simulink model "Modelo_global_NL_control_sobre_eje_q_2_c_VI"  (R2017a)
settings: Solver=VariableStepAuto  StartTime=0.0  StopTime=10.0  RelTol=1e-3
undefined symbols (not defined in the file): alfa_cu, beq, Cts, Jeq, LambdaM, Ld, Lq, Pp, Rs, Rsref, Rts, Tamb, Tsref
settings Model: Creator=merem  LastModifiedBy=merem

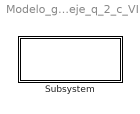
== system Modelo_global_NL_control_sobre_eje_q_2_c_VI ==
  Subsystem : Subsystem

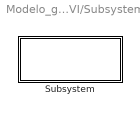
== system Modelo_global_NL_control_sobre_eje_q_2_c_VI/Subsystem ==
  Subsystem : Subsystem

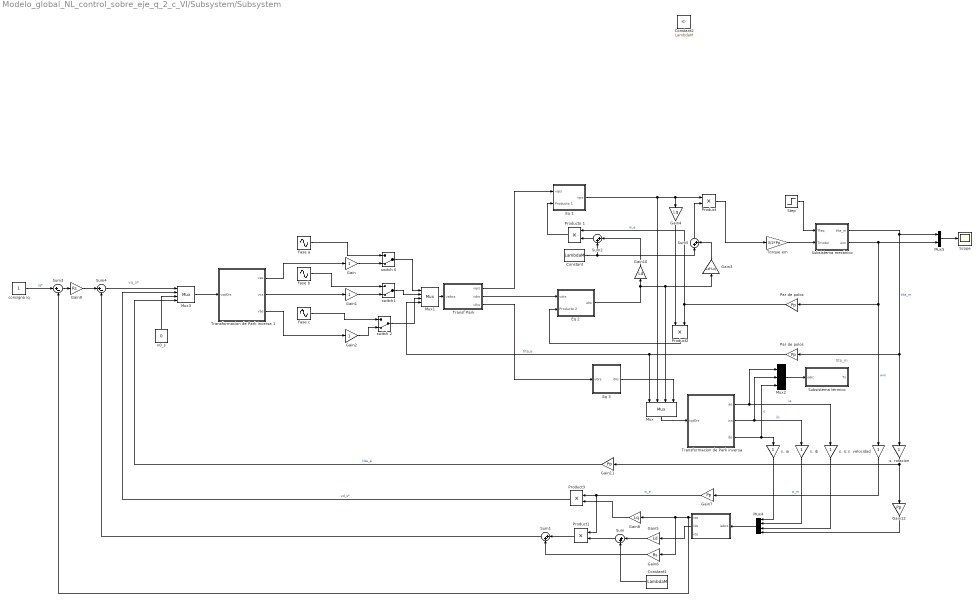
== system Modelo_global_NL_control_sobre_eje_q_2_c_VI/Subsystem/Subsystem ==
  note: vq_s*
  note: tita_m
  " " : Subsystem
  Constant : Constant  Value=LambdaM
  Constant1 : Constant  Value=LambdaM
  Constant2 : Constant  Value=LambdaM
  Eq 1 : Subsystem
  "Eq 2 " : Subsystem
  Eq 3 : Subsystem
  Fase a : Sin  SampleTime=0
  Fase b : Sin  SampleTime=0
  Fase c : Sin  SampleTime=0
  Gain : Gain
  Gain1 : Gain
  Gain10 : Gain  Gain=Ld
  Gain11 : Gain  Gain=Pp
  Gain12 : Gain  Gain=Pp
  Gain2 : Gain
  Gain3 : Gain  Gain=Ld-Lq
  Gain4 : Gain  Gain=Lq
  Gain5 : Gain  Gain=Ld
  Gain6 : Gain  Gain=Rs
  Gain7 : Gain  Gain=Pp
  Gain8 : Gain  Gain=Lq
  Gain9 : Gain  Gain=Rs
  Mux{,1,3..4} (4 alike) : Mux
      Mux settings: DisplayOption=signals
      Mux1 settings: DisplayOption=signals
      Mux3 settings: DisplayOption=signals
  Mux2 : Mux  Inputs=3
      settings: DisplayOption=signals
  Mux5 : Mux  Inputs=2
  Par de polos : Gain  Gain=Pp
  "Par de polos " : Gain  Gain=Pp
  Product{,1..3} (4 alike) : Product
  Producto 1 : Product
  Scope : Scope
  Step : Step  After=6.28  SampleTime=0
  Subsistema mecánico : Subsystem
  Subsistema térmico : Subsystem
  Sum{,1..2,5} (4 alike) : Sum  Inputs=|++
  Sum3 : Sum  Inputs=|+-
  Sum4 : Sum  Inputs=|+-
  "Torque em " : Gain  Gain=3/2*Pp
  "Transf Park " : Subsystem
  "Transformacion de Park inversa " : Subsystem
  Transformacion de Park inversa 1 : Subsystem
  consigna iq : Constant
  s. ia : Gain
  s. ib : Gain
  "s. ic " : Gain
  s. rotacion : Gain
  s. velocidad : Gain
  switch 0 : ManualSwitch  CurrentSetting=0
  "switch 2 " : ManualSwitch  CurrentSetting=0
  switch1 : ManualSwitch  CurrentSetting=0
  v0_s : Constant  Value=0
  wires:
  Product/1 -> "Torque em "/1
  Par de polos/1 -> Producto 1/1, Product2/2  "w_e"
  Sum2/1 -> Producto 1/2
  Gain10/1 -> Sum2/1
  Constant/1 -> Sum5/1, Sum2/2
  Sum5/1 -> Product/2
  Gain3/1 -> Sum5/2
  Gain4/1 -> Product2/1
  Eq 1/1("iqrs ") -> Gain4/1, Product/1, Mux/2
  Producto 1/1 -> Eq 1/2("Producto 1 ")
  "Eq 2 "/1("idrs ") -> Gain3/1, Mux/3, Gain10/1
  Product2/1 -> "Eq 2 "/2("Producto 2 ")
  Step/1 -> Subsistema mecánico/1("Tleq ")
  "Torque em "/1 -> Subsistema mecánico/2("Tmotor ")
  Subsistema mecánico/1("tita_m ") -> "Par de polos "/1, s. rotacion/1, Mux5/1  "tita_m"
  "Par de polos "/1 -> Mux/1, Mux1/4  "tita_e"
  "Transf Park "/2("vdrs ") -> "Eq 2 "/1("vdrs ")
  "Transf Park "/3("v0rs ") -> Eq 3/1("v0rs ")
  Mux/1 -> "Transformacion de Park inversa "/1(iqd0rs)
  Mux1/1 -> "Transf Park "/1("vabcs ")
  Eq 3/1("i0rs ") -> Mux/4
  switch 0/1 -> Mux1/1
  switch1/1 -> Mux1/2
  "switch 2 "/1 -> Mux1/3
  Gain/1 -> switch 0/2
  Gain1/1 -> switch1/2
  Gain2/1 -> "switch 2 "/2
  Transformacion de Park inversa 1/2("vcs ") -> Gain1/1
  Transformacion de Park inversa 1/3(vbs) -> Gain2/1
  Transformacion de Park inversa 1/1(vas) -> Gain/1
  Mux3/1 -> Transformacion de Park inversa 1/1(vqd0rs)
  "Transformacion de Park inversa "/3(ibs) -> Mux2/3, s. ia/1  "ic"
  "Transformacion de Park inversa "/2("ics ") -> Mux2/2, s. ib/1  "ib"
  "Transformacion de Park inversa "/1(ias) -> Mux2/1, "s. ic "/1  "ia"
  s. ia/1 -> Mux4/1
  s. ib/1 -> Mux4/2
  "s. ic "/1 -> Mux4/3
  Mux4/1 -> " "/1("iabcs ")
  " "/2("ids ") -> Gain5/1
  Gain5/1 -> Sum/1
  Constant1/1 -> Sum/2
  s. velocidad/1 -> Gain7/1  "w_m"
  Sum/1 -> Product1/2
  Product1/1 -> Sum1/1
  " "/1(iqs) -> Gain8/1, Gain6/1, Sum3/2
  Gain6/1 -> Sum1/2
  Gain7/1 -> Product3/1, Product1/1  "w_e"
  Gain8/1 -> Product3/2
  consigna iq/1 -> Sum3/1  "iq*"
  Sum3/1 -> Gain9/1
  Gain9/1 -> Sum4/1
  Sum1/1 -> Sum4/2
  Sum4/1 -> Mux3/1
  Product3/1 -> Mux3/2  "vd_s*"
  s. rotacion/1 -> Gain11/1, Gain12/1
  Gain11/1 -> Mux3/4  "tita_e"
  v0_s/1 -> Mux3/3
  Mux5/1 -> Scope/1
  Fase a/1 -> switch 0/1
  Fase b/1 -> switch1/1
  Fase c/1 -> "switch 2 "/1
  Mux2/1 -> Subsistema térmico/1(iabc)
  Subsistema mecánico/2("wm ") -> Par de polos/1, s. velocidad/1, Mux5/2  "wm"
  "Transf Park "/1(vqrs) -> Eq 1/1(vqrs)
  Gain12/1 -> Mux4/4

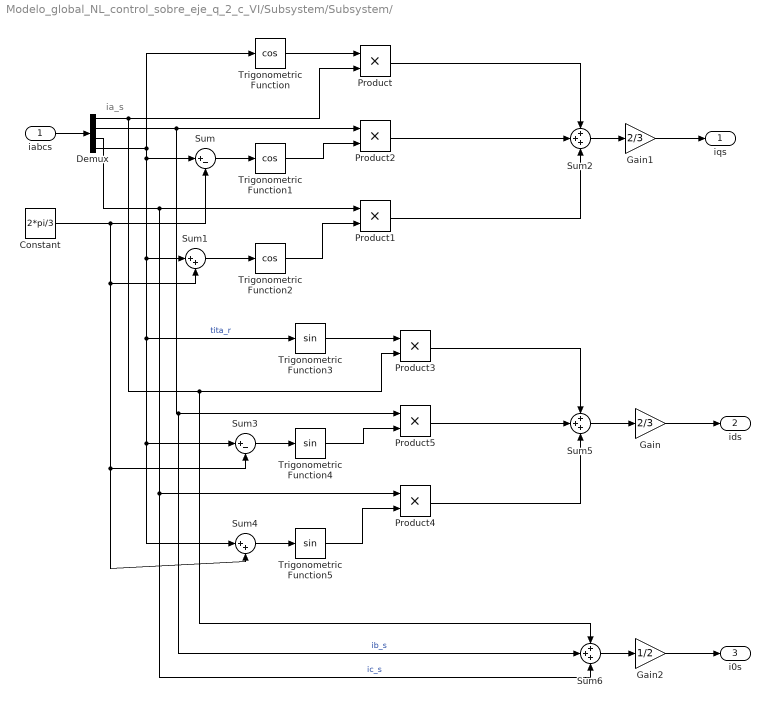
== system Modelo_global_NL_control_sobre_eje_q_2_c_VI/Subsystem/Subsystem/  ==
  note: ia_s
  "iabcs " : Inport
  Constant : Constant  Value=2*pi/3
  Demux : Demux
  Gain : Gain  Gain=2/3
  Gain1 : Gain  Gain=2/3
  Gain2 : Gain  Gain=1/2
  Product{,1..5} (6 alike) : Product
  Sum : Sum  Inputs=|+-
  Sum1 : Sum  Inputs=|++
  Sum2 : Sum  Inputs=+++
  Sum3 : Sum  Inputs=|+-
  Sum4 : Sum  Inputs=|++
  Sum5 : Sum  Inputs=+++
  Sum6 : Sum  Inputs=+++
  Trigonometric Function : Trigonometry  Operator=cos
  Trigonometric Function1 : Trigonometry  Operator=cos
  Trigonometric Function2 : Trigonometry  Operator=cos
  Trigonometric Function3 : Trigonometry
  Trigonometric Function4 : Trigonometry
  Trigonometric Function5 : Trigonometry
  iqs : Outport
  "ids " : Outport  Port=2
  "i0s " : Outport  Port=3
  wires:
  "iabcs "/1 -> Demux/1
  Demux/4 -> Sum1/1, Trigonometric Function3/1, Sum3/1, Sum4/1, Sum/1, Trigonometric Function/1  "tita_r"
  Trigonometric Function/1 -> Product/1
  Demux/1 -> Sum6/1, Product3/2, Product/2
  Constant/1 -> Sum4/2, Sum3/2, Sum1/2, Sum/2
  Sum/1 -> Trigonometric Function1/1
  Sum1/1 -> Trigonometric Function2/1
  Trigonometric Function1/1 -> Product2/2
  Trigonometric Function2/1 -> Product1/2
  Demux/2 -> Sum6/2, Product5/1, Product2/1  "ib_s"
  Demux/3 -> Sum6/3, Product4/1, Product1/1  "ic_s"
  Product/1 -> Sum2/1
  Product2/1 -> Sum2/2
  Sum2/1 -> Gain1/1
  Trigonometric Function5/1 -> Product4/2
  Trigonometric Function3/1 -> Product3/1
  Sum4/1 -> Trigonometric Function5/1
  Sum3/1 -> Trigonometric Function4/1
  Trigonometric Function4/1 -> Product5/2
  Product3/1 -> Sum5/1
  Product5/1 -> Sum5/2
  Product4/1 -> Sum5/3
  Sum5/1 -> Gain/1
  Product1/1 -> Sum2/3
  Gain/1 -> "ids "/1
  Gain1/1 -> iqs/1
  Sum6/1 -> Gain2/1
  Gain2/1 -> "i0s "/1

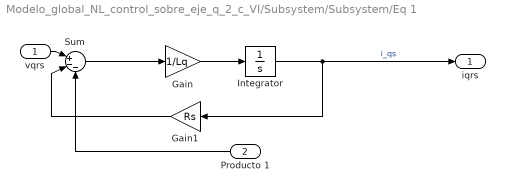
== system Modelo_global_NL_control_sobre_eje_q_2_c_VI/Subsystem/Subsystem/Eq 1 ==
  vqrs : Inport
  "Producto 1 " : Inport  Port=2
  Gain : Gain  Gain=1/Lq
  Gain1 : Gain  Gain=Rs
  Integrator : Integrator
  Sum : Sum  Inputs=|+--
  "iqrs " : Outport
  wires:
  Gain/1 -> Integrator/1
  Sum/1 -> Gain/1
  vqrs/1 -> Sum/1
  Gain1/1 -> Sum/2
  "Producto 1 "/1 -> Sum/3
  Integrator/1 -> "iqrs "/1, Gain1/1  "i_qs"

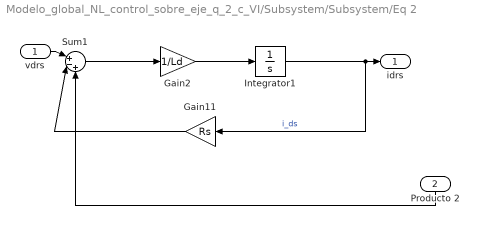
== system Modelo_global_NL_control_sobre_eje_q_2_c_VI/Subsystem/Subsystem/Eq 2  ==
  "vdrs " : Inport
  "Producto 2 " : Inport  Port=2
  Gain11 : Gain  Gain=Rs
  Gain2 : Gain  Gain=1/Ld
  Integrator1 : Integrator
  Sum1 : Sum  Inputs=|+-+
  "idrs " : Outport
  wires:
  "Producto 2 "/1 -> Sum1/3
  Gain2/1 -> Integrator1/1
  Gain11/1 -> Sum1/2
  Sum1/1 -> Gain2/1
  Integrator1/1 -> Gain11/1, "idrs "/1  "i_ds"
  "vdrs "/1 -> Sum1/1

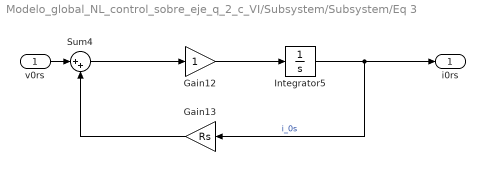
== system Modelo_global_NL_control_sobre_eje_q_2_c_VI/Subsystem/Subsystem/Eq 3 ==
  "v0rs " : Inport
  Gain12 : Gain
  Gain13 : Gain  Gain=Rs
  Integrator5 : Integrator
  Sum4 : Sum  Inputs=|++
  "i0rs " : Outport
  wires:
  Gain12/1 -> Integrator5/1
  Sum4/1 -> Gain12/1
  Gain13/1 -> Sum4/2
  "v0rs "/1 -> Sum4/1
  Integrator5/1 -> "i0rs "/1, Gain13/1  "i_0s"

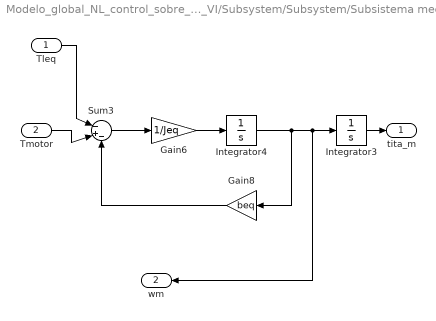
== system Modelo_global_NL_control_sobre_eje_q_2_c_VI/Subsystem/Subsystem/Subsistema mecánico ==
  "Tleq " : Inport
  "Tmotor " : Inport  Port=2
  Gain6 : Gain  Gain=1/Jeq
  Gain8 : Gain  Gain=beq
  Integrator3 : Integrator
  Integrator4 : Integrator
  Sum3 : Sum  Inputs=|-+-
  "tita_m " : Outport
  "wm " : Outport  Port=2
  wires:
  Integrator3/1 -> "tita_m "/1
  Integrator4/1 -> Gain8/1, "wm "/1, Integrator3/1
  Sum3/1 -> Gain6/1
  Gain6/1 -> Integrator4/1
  Gain8/1 -> Sum3/3
  "Tleq "/1 -> Sum3/1
  "Tmotor "/1 -> Sum3/2

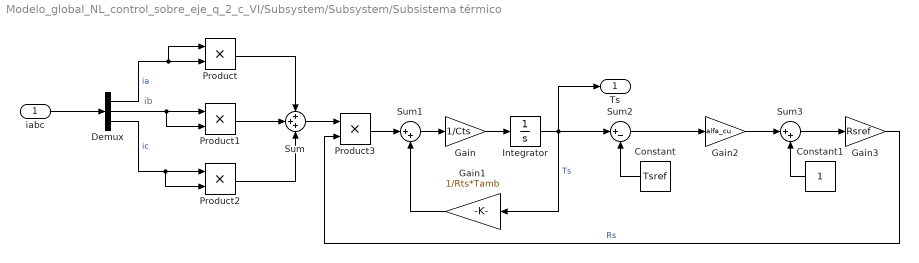
== system Modelo_global_NL_control_sobre_eje_q_2_c_VI/Subsystem/Subsystem/Subsistema térmico ==
  note: ib
  iabc : Inport
  Constant : Constant  Value=Tsref
  Constant1 : Constant
  Demux : Demux  Outputs=3
  Gain : Gain  Gain=1/Cts
  Gain1 : Gain  Gain=1/Rts*Tamb
  Gain2 : Gain  Gain=alfa_cu
  Gain3 : Gain  Gain=Rsref
  Integrator : Integrator
  Product{,1..3} (4 alike) : Product
  Sum : Sum  Inputs=+++
  Sum1 : Sum  Inputs=|++
  Sum2 : Sum  Inputs=|+-
  Sum3 : Sum  Inputs=|++
  Ts : Outport
  wires:
  iabc/1 -> Demux/1
  Demux/1 -> Product/2, Product/1  "ia"
  Demux/2 -> Product1/2, Product1/1
  Demux/3 -> Product2/2, Product2/1  "ic"
  Product/1 -> Sum/1
  Product1/1 -> Sum/2
  Product2/1 -> Sum/3
  Sum/1 -> Product3/1
  Gain/1 -> Integrator/1
  Product3/1 -> Sum1/1
  Sum1/1 -> Gain/1
  Gain1/1 -> Sum1/2
  Integrator/1 -> Ts/1, Sum2/1, Gain1/1  "Ts"
  Constant/1 -> Sum2/2
  Sum2/1 -> Gain2/1
  Gain2/1 -> Sum3/1
  Constant1/1 -> Sum3/2
  Sum3/1 -> Gain3/1
  Gain3/1 -> Product3/2  "Rs"

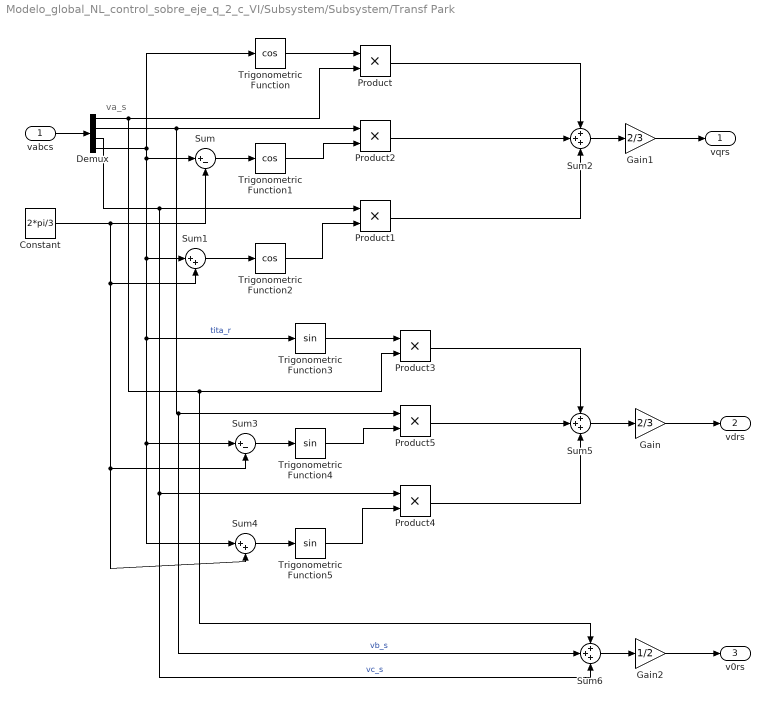
== system Modelo_global_NL_control_sobre_eje_q_2_c_VI/Subsystem/Subsystem/Transf Park  ==
  note: va_s
  "vabcs " : Inport
  Constant : Constant  Value=2*pi/3
  Demux : Demux
  Gain : Gain  Gain=2/3
  Gain1 : Gain  Gain=2/3
  Gain2 : Gain  Gain=1/2
  Product{,1..5} (6 alike) : Product
  Sum : Sum  Inputs=|+-
  Sum1 : Sum  Inputs=|++
  Sum2 : Sum  Inputs=+++
  Sum3 : Sum  Inputs=|+-
  Sum4 : Sum  Inputs=|++
  Sum5 : Sum  Inputs=+++
  Sum6 : Sum  Inputs=+++
  Trigonometric Function : Trigonometry  Operator=cos
  Trigonometric Function1 : Trigonometry  Operator=cos
  Trigonometric Function2 : Trigonometry  Operator=cos
  Trigonometric Function3 : Trigonometry
  Trigonometric Function4 : Trigonometry
  Trigonometric Function5 : Trigonometry
  vqrs : Outport
  "vdrs " : Outport  Port=2
  "v0rs " : Outport  Port=3
  wires:
  "vabcs "/1 -> Demux/1
  Demux/4 -> Sum1/1, Trigonometric Function3/1, Sum3/1, Sum4/1, Sum/1, Trigonometric Function/1  "tita_r"
  Trigonometric Function/1 -> Product/1
  Demux/1 -> Sum6/1, Product3/2, Product/2
  Constant/1 -> Sum4/2, Sum3/2, Sum1/2, Sum/2
  Sum/1 -> Trigonometric Function1/1
  Sum1/1 -> Trigonometric Function2/1
  Trigonometric Function1/1 -> Product2/2
  Trigonometric Function2/1 -> Product1/2
  Demux/2 -> Sum6/2, Product5/1, Product2/1  "vb_s"
  Demux/3 -> Sum6/3, Product4/1, Product1/1  "vc_s"
  Product/1 -> Sum2/1
  Product2/1 -> Sum2/2
  Sum2/1 -> Gain1/1
  Trigonometric Function5/1 -> Product4/2
  Trigonometric Function3/1 -> Product3/1
  Sum4/1 -> Trigonometric Function5/1
  Sum3/1 -> Trigonometric Function4/1
  Trigonometric Function4/1 -> Product5/2
  Product3/1 -> Sum5/1
  Product5/1 -> Sum5/2
  Product4/1 -> Sum5/3
  Sum5/1 -> Gain/1
  Product1/1 -> Sum2/3
  Gain/1 -> "vdrs "/1
  Gain1/1 -> vqrs/1
  Sum6/1 -> Gain2/1
  Gain2/1 -> "v0rs "/1

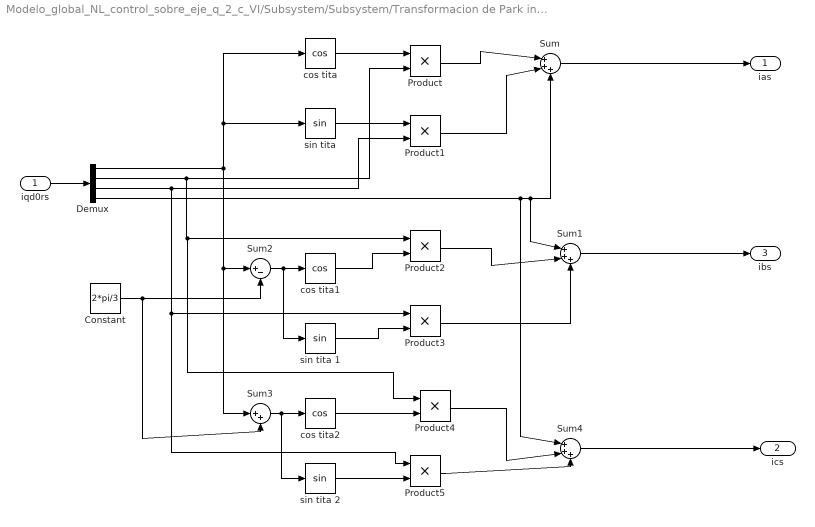
== system Modelo_global_NL_control_sobre_eje_q_2_c_VI/Subsystem/Subsystem/Transformacion de Park inversa  ==
  iqd0rs : Inport
  Constant : Constant  Value=2*pi/3
  Demux : Demux
  Product{,1..5} (6 alike) : Product
  Sum : Sum  Inputs=|+++
  Sum1 : Sum  Inputs=|+++
  Sum2 : Sum  Inputs=|+-
  Sum3 : Sum  Inputs=|++
  Sum4 : Sum  Inputs=|+++
  cos tita : Trigonometry  Operator=cos
  cos tita1 : Trigonometry  Operator=cos
  cos tita2 : Trigonometry  Operator=cos
  "sin tita " : Trigonometry
  sin tita 1 : Trigonometry
  sin tita 2 : Trigonometry
  ias : Outport
  "ics " : Outport  Port=2
  ibs : Outport  Port=3
  wires:
  iqd0rs/1 -> Demux/1
  Demux/1 -> Sum3/1, Sum2/1, cos tita/1, "sin tita "/1
  Demux/2 -> Product4/1, Product2/1, Product/2
  cos tita/1 -> Product/1
  "sin tita "/1 -> Product1/1
  Demux/3 -> Product5/1, Product3/1, Product1/2
  Product/1 -> Sum/1
  Product1/1 -> Sum/2
  Sum/1 -> ias/1
  Demux/4 -> Sum4/1, Sum1/1, Sum/3
  cos tita1/1 -> Product2/2
  sin tita 1/1 -> Product3/2
  Product3/1 -> Sum1/3
  Product2/1 -> Sum1/2
  Sum1/1 -> ibs/1
  Constant/1 -> Sum3/2, Sum2/2
  Sum2/1 -> sin tita 1/1, cos tita1/1
  Sum3/1 -> sin tita 2/1, cos tita2/1
  cos tita2/1 -> Product4/2
  sin tita 2/1 -> Product5/2
  Product5/1 -> Sum4/3
  Product4/1 -> Sum4/2
  Sum4/1 -> "ics "/1

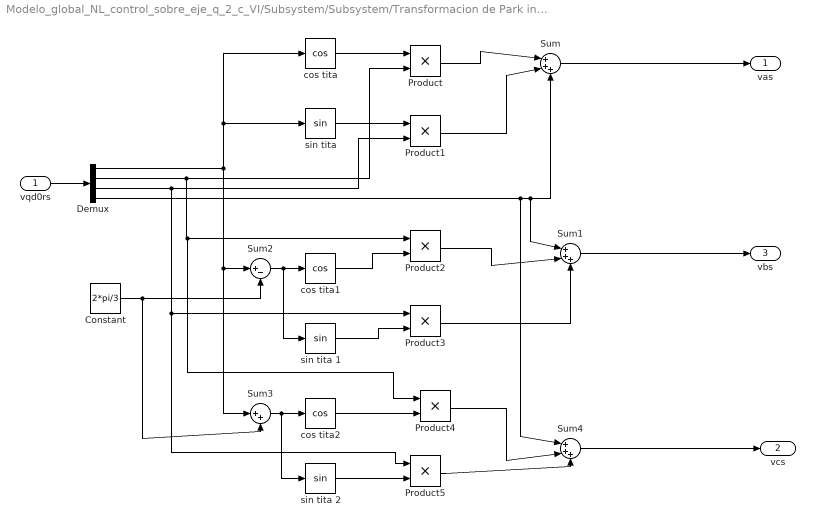
== system Modelo_global_NL_control_sobre_eje_q_2_c_VI/Subsystem/Subsystem/Transformacion de Park inversa 1 ==
  vqd0rs : Inport
  Constant : Constant  Value=2*pi/3
  Demux : Demux
  Product{,1..5} (6 alike) : Product
  Sum : Sum  Inputs=|+++
  Sum1 : Sum  Inputs=|+++
  Sum2 : Sum  Inputs=|+-
  Sum3 : Sum  Inputs=|++
  Sum4 : Sum  Inputs=|+++
  cos tita : Trigonometry  Operator=cos
  cos tita1 : Trigonometry  Operator=cos
  cos tita2 : Trigonometry  Operator=cos
  "sin tita " : Trigonometry
  sin tita 1 : Trigonometry
  sin tita 2 : Trigonometry
  vas : Outport
  "vcs " : Outport  Port=2
  vbs : Outport  Port=3
  wires:
  vqd0rs/1 -> Demux/1
  Demux/1 -> Sum3/1, Sum2/1, cos tita/1, "sin tita "/1
  Demux/2 -> Product4/1, Product2/1, Product/2
  cos tita/1 -> Product/1
  "sin tita "/1 -> Product1/1
  Demux/3 -> Product5/1, Product3/1, Product1/2
  Product/1 -> Sum/1
  Product1/1 -> Sum/2
  Sum/1 -> vas/1
  Demux/4 -> Sum4/1, Sum1/1, Sum/3
  cos tita1/1 -> Product2/2
  sin tita 1/1 -> Product3/2
  Product3/1 -> Sum1/3
  Product2/1 -> Sum1/2
  Sum1/1 -> vbs/1
  Constant/1 -> Sum3/2, Sum2/2
  Sum2/1 -> sin tita 1/1, cos tita1/1
  Sum3/1 -> sin tita 2/1, cos tita2/1
  cos tita2/1 -> Product4/2
  sin tita 2/1 -> Product5/2
  Product5/1 -> Sum4/3
  Product4/1 -> Sum4/2
  Sum4/1 -> "vcs "/1
